simulink model "LAB1"  (R2023a)
settings: Solver=VariableStepAuto  StartTime=0.0  StopTime=10.0  MaxStep=0.01  RelTol=1e-3
settings Model: Creator=Mohamed Ezzelrgal  LastModifiedBy=Mohamed Ezzelrgal

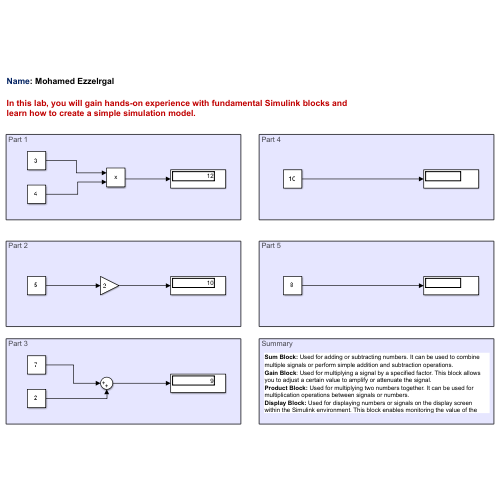
[thumbnail: Simulink's stored preview of the top-level diagram]
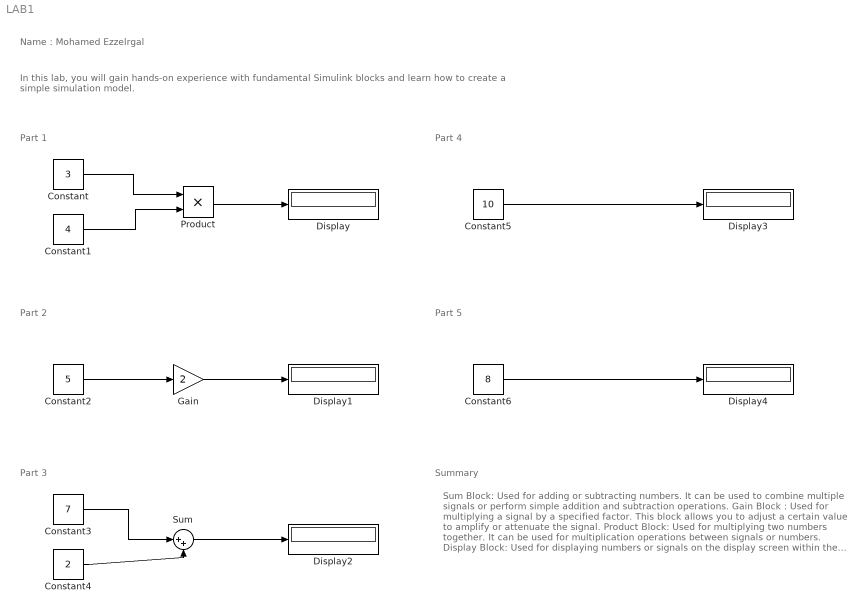
== system LAB1 ==
  note: Name : Mohamed Ezzelrgal
  note: In this lab, you will gain hands-on experience with fundamental Simulink blocks and learn how to create a simple simulation model.
  note: Sum Block: Used for adding or subtracting numbers. It can be used to combine multiple signals or perform simple addition and subtraction operations.
      | Gain Block : Used for multiplying a signal by a specified factor. This block allows you to adjust a certain value to amplify or attenuate the signal.
      | Product Block: Used for multiplying two numbers together. It can be used for multiplication operations between signals or numbers.
      | Display Block: Used for displaying numbers or signals on the display screen within the Simulink environment. This block enables monitoring the value of the signal or numbers during model execution.
  note: Part 1
  note: Part 2
  note: Part 3
  note: Part 4
  note: Part 5
  note: Summary
  Constant : Constant  Value=3
  Constant1 : Constant  Value=4
  Constant2 : Constant  Value=5
  Constant3 : Constant  Value=7
  Constant4 : Constant  Value=2
  Constant5 : Constant  Value=10
  Constant6 : Constant  Value=8
  Display{,1..4} (5 alike) : Display
      Display3 settings: Decimation=2
      Display4 settings: Decimation=2
  Gain : Gain  Gain=2
  Product : Product
  Sum : Sum  Inputs=|++
  wires:
  Constant/1 -> Product/1
  Constant1/1 -> Product/2
  Product/1 -> Display/1
  Constant2/1 -> Gain/1
  Gain/1 -> Display1/1
  Constant4/1 -> Sum/2
  Constant3/1 -> Sum/1
  Sum/1 -> Display2/1
  Constant5/1 -> Display3/1
  Constant6/1 -> Display4/1
